simulink model "MEEN_432_Proj4Part2_version2025A"  (R2025a)
settings: Solver=VariableStepAuto  StartTime=0.0  StopTime=3600  FixedStep=0.01  RelTol=1e-3
undefined symbols (not defined in the file): carData, datBat, datCar, datMotor
libraries: slpidlib x1
settings Model: Creator=dxego  LastModifiedBy=jthin
settings OptimizationCC: ReuseModelBlockBuffer=off
settings RTWCC: GPUComputeCapability=3.5

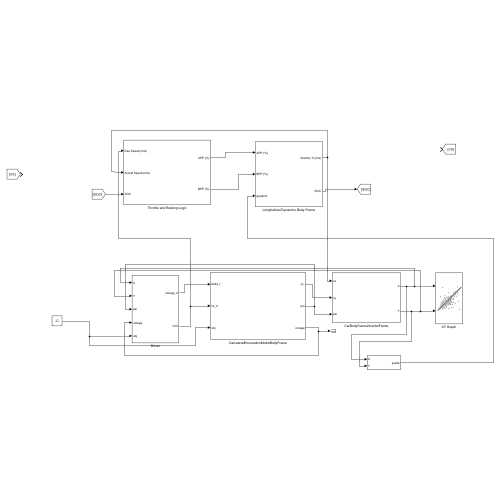
[thumbnail: Simulink's stored preview of the top-level diagram]
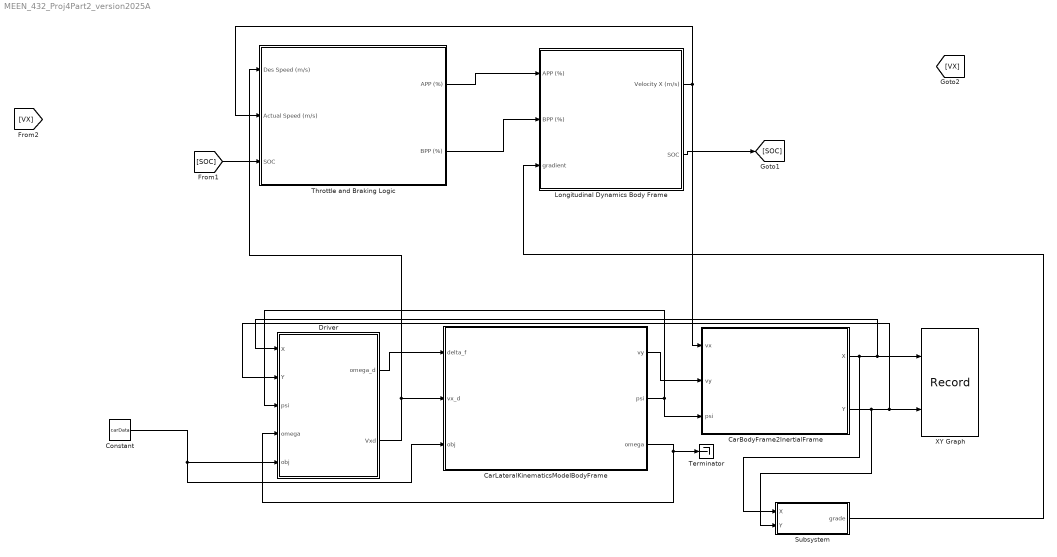
== system MEEN_432_Proj4Part2_version2025A ==
  CarBodyFrame2InertialFrame : Subsystem
  CarLateralKinematicsModelBodyFrame : Subsystem
  Constant : Constant  Value=carData  OutDataTypeStr=Bus: slBus1
  Driver : Subsystem
  Longitudinal Dynamics Body Frame : Subsystem
  Subsystem : Subsystem
  Terminator : Terminator
  "Throttle and Braking Logic " : Subsystem
  XY Graph : Record  NumPorts=2.0  FileSettingsInternal="{\"entries\":[{\"content\":{\"excelSettings\":{\"content\":{},\"type\":\"Streamout.ExcelSettings\"},\"parquetSettings\":{\"content\":{},\"type\":\"Streamout.ParquetSettings\"}},\"type\":\"Streamout.FileSettingStorage\",\"uuid\":\"\"}],\"packageUris\":[\"http:\\/\\/schema.mathworks.com\\/mf0\\/streamout_blocks\\/R2020a\"],\"version\":\"1.0\"}"  FrameSettings=[0, 0]  Layout=[1 1]  SignalsInternal="{\"entries\":[{\"content\":{\"signals\":[{\"content\":{\"blockPath\":[],\"dimensions\":[1],\"domain\":\"\",\"lineColor\":\"#a2142f\",\"plots\":[ 1 ],\"port\":1,\"signalID\":1,\"signalName\":\"CarBodyFrame2InertialFrame:1\"},\"type\":\"RecordBlkView.Signal\",\"uuid\":\"\"},{\"content\":{\"blockPath\":[],\"dimensions\":[1],\"domain\":\"\",\"lineColor\":\"#139fff\",\"plots\":[ 1 ],\"port\":2,\"signalID\":2,\"signalName\":\"CarBodyFrame2InertialFrame:2\"},\"type\":\"RecordBlkView.Signal\",\"uuid\":\"\"}]},\"type\":\"RecordBlkView.InputSignals\",\"uuid\":\"\"}],\"packageUris\":[\"http:\\/\\/schema.mathworks.com\\/mf0\\/streamout_blocks\\/R2020a\"],\"version\":\"1.0\"}"  VisualizationBindings="{\"xyplotplugin\":{\"info\":[{\"series\":[{\"bindingParametersList\":[{\"parameter\":\"X-Axis\",\"signalID\":1,\"signalName\":\"CarBodyFrame2InertialFrame:1\"},{\"parameter\":\"Y-Axis\",\"signalID\":2,\"signalName\":\"CarBodyFrame2InertialFrame:2\"}],\"seriesID\":0}],\"subplotID\":1}]}}"  CompatibilityTag=XY  st=-1
  wires:
  "Throttle and Braking Logic "/1(APP (%)) -> Longitudinal Dynamics Body Frame/1(APP (%))
  "Throttle and Braking Logic "/2(BPP (%)) -> Longitudinal Dynamics Body Frame/2("BPP (%) ")
  Longitudinal Dynamics Body Frame/2(SOC) -> [SOC]
  [SOC] -> "Throttle and Braking Logic "/3(SOC)
  CarLateralKinematicsModelBodyFrame/1("vy ") -> CarBodyFrame2InertialFrame/2(vy)
  Driver/1(omega_d) -> CarLateralKinematicsModelBodyFrame/1(delta_f)
  Constant/1 -> CarLateralKinematicsModelBodyFrame/3(obj), Driver/5(obj)
  CarBodyFrame2InertialFrame/2(Y) -> Subsystem/2(Y), Driver/2(Y), XY Graph/2
  CarLateralKinematicsModelBodyFrame/2(psi) -> CarBodyFrame2InertialFrame/3(psi), Driver/3(psi)
  CarBodyFrame2InertialFrame/1(X) -> Subsystem/1(X), Driver/1(X), XY Graph/1
  CarLateralKinematicsModelBodyFrame/3(omega) -> Driver/4(omega), Terminator/1
  Driver/2(Vxd) -> "Throttle and Braking Logic "/1("Des Speed (m/s) "), CarLateralKinematicsModelBodyFrame/2("vx_d ")
  Longitudinal Dynamics Body Frame/1(Velocity X (m/s)) -> "Throttle and Braking Logic "/2(Actual Speed (m/s)), CarBodyFrame2InertialFrame/1(vx)
  Subsystem/1(grade) -> Longitudinal Dynamics Body Frame/3(gradient)

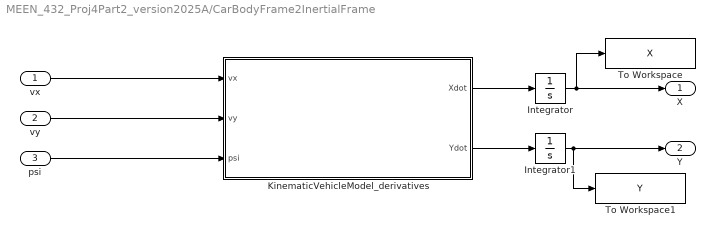
== system MEEN_432_Proj4Part2_version2025A/CarBodyFrame2InertialFrame ==
  vx : Inport
  vy : Inport  Port=2
  psi : Inport  Port=3
  Integrator : Integrator  InitialCondition=carData.init.X0
  Integrator1 : Integrator  InitialCondition=carData.init.Y0
  KinematicVehicleModel_derivatives : MATLAB Function  TreatAsAtomicUnit=on
  To Workspace : ToWorkspace  VariableName=X  SaveFormat=Timeseries  SampleTime=-1
  To Workspace1 : ToWorkspace  VariableName=Y  SaveFormat=Timeseries  SampleTime=-1
  X : Outport
  Y : Outport  Port=2
  wires:
  KinematicVehicleModel_derivatives/1(Xdot) -> Integrator/1
  KinematicVehicleModel_derivatives/2(Ydot) -> Integrator1/1
  Integrator/1 -> To Workspace/1, X/1
  Integrator1/1 -> To Workspace1/1, Y/1
  vx/1 -> KinematicVehicleModel_derivatives/1(vx)
  vy/1 -> KinematicVehicleModel_derivatives/2(vy)
  psi/1 -> KinematicVehicleModel_derivatives/3(psi)

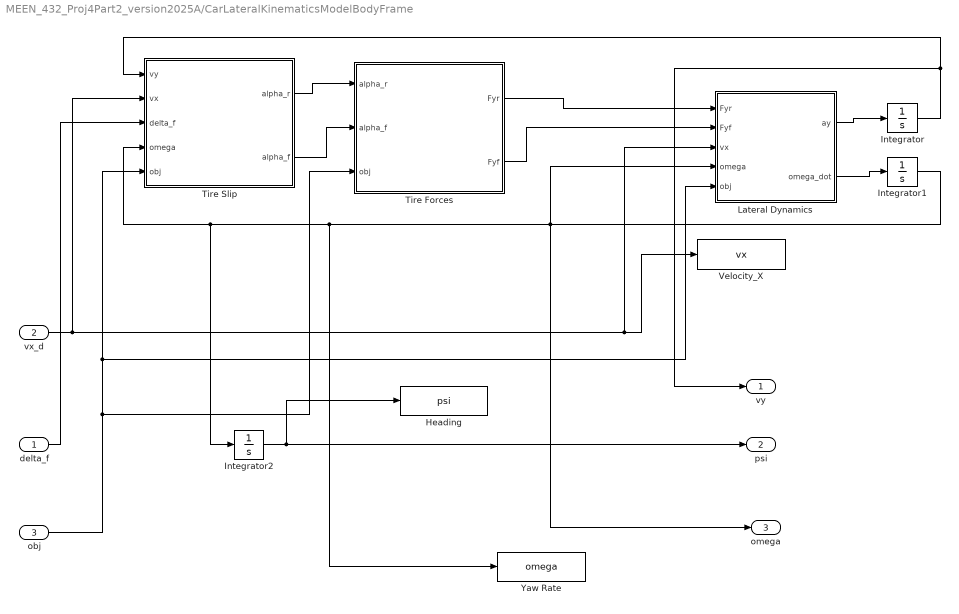
== system MEEN_432_Proj4Part2_version2025A/CarLateralKinematicsModelBodyFrame ==
  delta_f : Inport
  "vx_d " : Inport  Port=2
  obj : Inport  Port=3
  Heading : ToWorkspace  VariableName=psi  SaveFormat=Timeseries  SampleTime=-1
  Integrator : Integrator
  Integrator1 : Integrator
  Integrator2 : Integrator
  Lateral Dynamics : MATLAB Function  TreatAsAtomicUnit=on
  Tire Forces : MATLAB Function  TreatAsAtomicUnit=on
  Tire Slip : MATLAB Function  TreatAsAtomicUnit=on
  Velocity_X : ToWorkspace  VariableName=vx  SaveFormat=Timeseries  SampleTime=-1
  Yaw Rate : ToWorkspace  VariableName=omega  SaveFormat=Timeseries  SampleTime=-1
  "vy " : Outport
  psi : Outport  Port=2
  omega : Outport  Port=3
  wires:
  Integrator2/1 -> psi/1, Heading/1
  "vx_d "/1 -> Tire Slip/2(vx), Velocity_X/1, Lateral Dynamics/3(vx)
  delta_f/1 -> Tire Slip/3(delta_f)
  Integrator/1 -> "vy "/1, Tire Slip/1(vy)
  Tire Slip/1(alpha_r) -> Tire Forces/1(alpha_r)
  Tire Slip/2(alpha_f) -> Tire Forces/2(alpha_f)
  Lateral Dynamics/1(ay) -> Integrator/1
  Lateral Dynamics/2(omega_dot) -> Integrator1/1
  Integrator1/1 -> omega/1, Lateral Dynamics/4(omega), Yaw Rate/1, Integrator2/1, Tire Slip/4(omega)
  Tire Forces/1(Fyr) -> Lateral Dynamics/1(Fyr)
  Tire Forces/2(Fyf) -> Lateral Dynamics/2(Fyf)
  obj/1 -> Tire Forces/3(obj), Lateral Dynamics/5(obj), Tire Slip/5(obj)

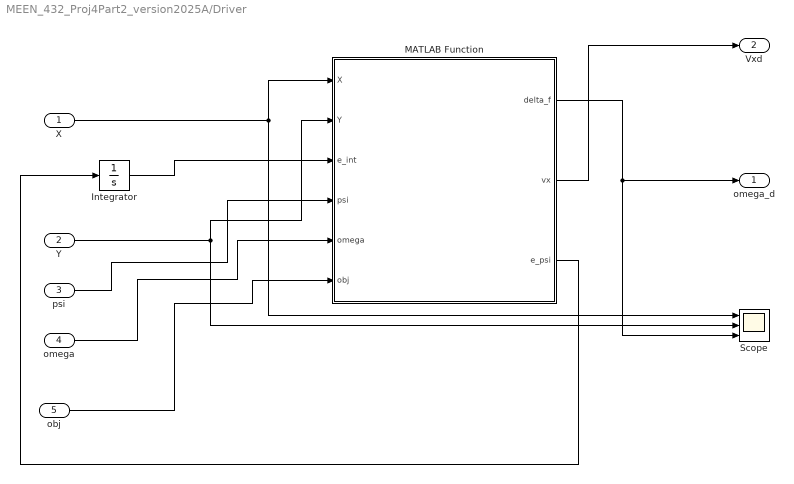
== system MEEN_432_Proj4Part2_version2025A/Driver ==
  X : Inport
  Y : Inport  Port=2
  psi : Inport  Port=3
  omega : Inport  Port=4
  obj : Inport  Port=5
  Integrator : Integrator
  MATLAB Function : MATLAB Function  TreatAsAtomicUnit=on
  Scope : Scope  NumInputPorts=3
      settings: ActiveDisplayYMinimum=-351.50186  ActiveDisplayYMaximum=1255.09761
  omega_d : Outport
  Vxd : Outport  Port=2
  wires:
  MATLAB Function/1(delta_f) -> omega_d/1, Scope/3
  MATLAB Function/2(vx) -> Vxd/1
  X/1 -> Scope/1, MATLAB Function/1(X)
  Y/1 -> Scope/2, MATLAB Function/2(Y)
  omega/1 -> MATLAB Function/5(omega)
  obj/1 -> MATLAB Function/6(obj)
  psi/1 -> MATLAB Function/4(psi)
  Integrator/1 -> MATLAB Function/3(e_int)
  MATLAB Function/3(e_psi) -> Integrator/1

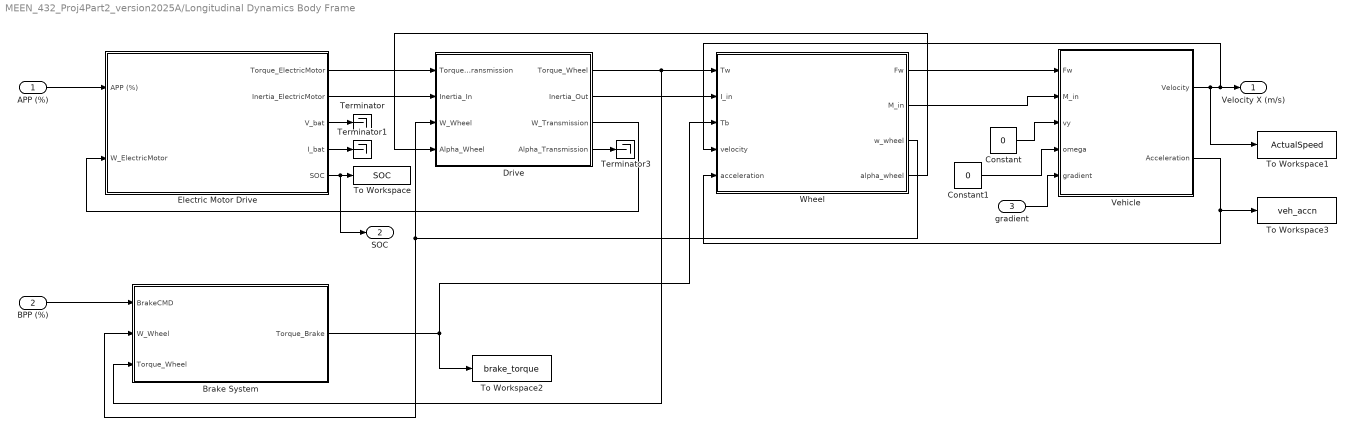
== system MEEN_432_Proj4Part2_version2025A/Longitudinal Dynamics Body Frame ==
  APP (%) : Inport
  "BPP (%) " : Inport  Port=2
  gradient : Inport  Port=3
  Brake System : Subsystem
  Constant : Constant  Value=0
  Constant1 : Constant  Value=0
  Drive : Subsystem
  Electric Motor Drive : Subsystem
  Terminator : Terminator
  Terminator1 : Terminator
  Terminator3 : Terminator
  To Workspace : ToWorkspace  VariableName=SOC  SaveFormat=Timeseries  SampleTime=-1
  To Workspace1 : ToWorkspace  VariableName=ActualSpeed  SaveFormat=Timeseries  SampleTime=-1
  To Workspace2 : ToWorkspace  VariableName=brake_torque  SaveFormat=Timeseries  SampleTime=-1
  To Workspace3 : ToWorkspace  VariableName=veh_accn  SaveFormat=Timeseries  SampleTime=-1
  Vehicle : Subsystem
  "Wheel " : Subsystem
  Velocity X (m/s) : Outport
  SOC : Outport  Port=2
  wires:
  Drive/3(W_Transmission) -> Electric Motor Drive/2(W_ElectricMotor)
  Electric Motor Drive/2(Inertia_ElectricMotor) -> Drive/2(Inertia_In)
  Electric Motor Drive/3(V_bat) -> Terminator/1
  Vehicle/2(Acceleration) -> "Wheel "/5(acceleration), To Workspace3/1
  Drive/1(Torque_Wheel) -> "Wheel "/1(Tw), Brake System/3(Torque_Wheel)
  Electric Motor Drive/1(Torque_ElectricMotor) -> Drive/1(Torque_Transmission)
  Drive/2(Inertia_Out) -> "Wheel "/2(I_in)
  "Wheel "/2(M_in) -> Vehicle/2("M_in ")
  "BPP (%) "/1 -> Brake System/1("BrakeCMD ")
  "Wheel "/3(w_wheel) -> Brake System/2(W_Wheel), Drive/3(W_Wheel)
  "Wheel "/1(Fw) -> Vehicle/1("Fw ")
  Brake System/1(Torque_Brake) -> To Workspace2/1, "Wheel "/3(Tb)
  Drive/4(Alpha_Transmission) -> Terminator3/1
  "Wheel "/4(alpha_wheel) -> Drive/4(Alpha_Wheel)
  Electric Motor Drive/4(I_bat) -> Terminator1/1
  APP (%)/1 -> Electric Motor Drive/1(APP (%))
  Constant/1 -> Vehicle/3(vy)
  Constant1/1 -> Vehicle/4(omega)
  Vehicle/1("Velocity ") -> To Workspace1/1, "Wheel "/4(velocity), Velocity X (m/s)/1
  Electric Motor Drive/5(SOC) -> SOC/1, To Workspace/1
  gradient/1 -> Vehicle/5(gradient)

== system MEEN_432_Proj4Part2_version2025A/Subsystem ==
  X : Inport
  Y : Inport  Port=2
  MATLAB Function : MATLAB Function  TreatAsAtomicUnit=on
  grade : Outport
  wires:
  X/1 -> MATLAB Function/1(X)
  Y/1 -> MATLAB Function/2(Y)
  MATLAB Function/1(calculate_gradient) -> grade/1

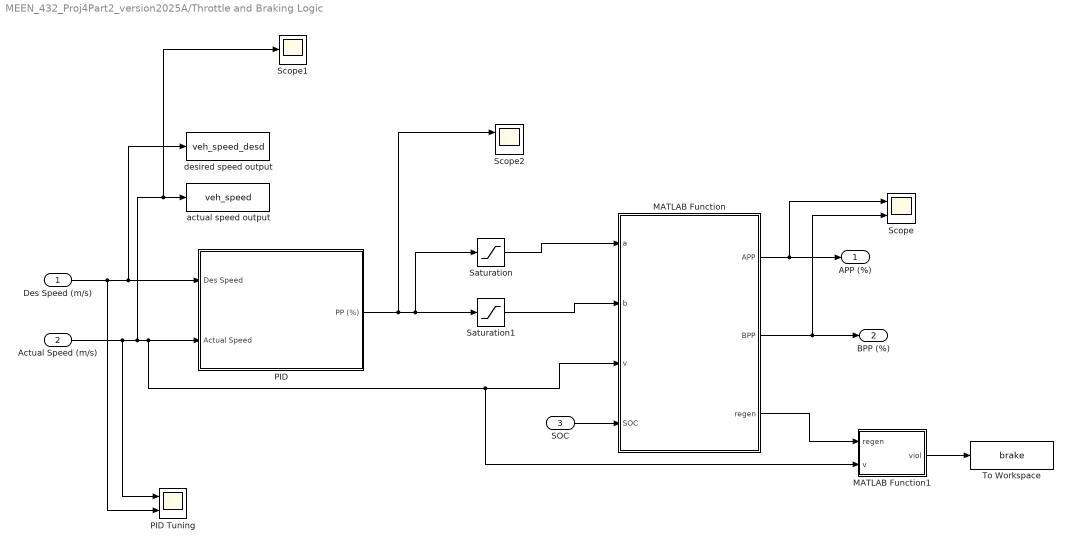
== system MEEN_432_Proj4Part2_version2025A/Throttle and Braking Logic  ==
  "Des Speed (m/s) " : Inport
  Actual Speed (m/s) : Inport  Port=2
  SOC : Inport  Port=3
  MATLAB Function : MATLAB Function  TreatAsAtomicUnit=on
  MATLAB Function1 : MATLAB Function  TreatAsAtomicUnit=on
  PID : Subsystem
  PID Tuning : Scope  NumInputPorts=2
      settings: ActiveDisplayYMinimum=-4.40832  ActiveDisplayYMaximum=37.63006
  Saturation : Saturate  UpperLimit=1  LowerLimit=0
  Saturation1 : Saturate  UpperLimit=0  LowerLimit=-1
  Scope : Scope  NumInputPorts=2
      settings: ActiveDisplayYMinimum=-1.0607  ActiveDisplayYMaximum=1.06103
  Scope1 : Scope
      settings: ActiveDisplayYMinimum=-3.08288  ActiveDisplayYMaximum=27.75461
  Scope2 : Scope  NumInputPorts=2
      settings: ActiveDisplayYMinimum=-1.0607  ActiveDisplayYMaximum=1.06103  DataLoggingVariableName=ScopeData5
  To Workspace : ToWorkspace  VariableName=brake  SaveFormat=Timeseries  SampleTime=-1
  actual speed output : ToWorkspace  VariableName=veh_speed  SaveFormat=Timeseries  SampleTime=-1
  desired speed output : ToWorkspace  VariableName=veh_speed_desd  SaveFormat=Timeseries  SampleTime=-1
  APP (%) : Outport
  BPP (%) : Outport  Port=2
  wires:
  PID/1(PP (%)) -> Scope2/1, Saturation1/1, Saturation/1
  Saturation1/1 -> MATLAB Function/2(b)
  Actual Speed (m/s)/1 -> PID Tuning/1, Scope1/1, actual speed output/1, MATLAB Function1/2(v), MATLAB Function/3(v), PID/2(Actual Speed)
  "Des Speed (m/s) "/1 -> PID Tuning/2, desired speed output/1, PID/1("Des Speed ")
  Saturation/1 -> MATLAB Function/1(a)
  MATLAB Function/1(APP) -> Scope/1, APP (%)/1
  MATLAB Function/2(BPP) -> Scope/2, BPP (%)/1
  MATLAB Function1/1(viol) -> To Workspace/1
  SOC/1 -> MATLAB Function/4(SOC)
  MATLAB Function/3(regen) -> MATLAB Function1/1(regen)

== system MEEN_432_Proj4Part2_version2025A/Longitudinal Dynamics Body Frame/Brake System ==
  "BrakeCMD " : Inport
  W_Wheel : Inport  Port=2
  Torque_Wheel : Inport  Port=3
  Brake Torque : MATLAB Function  TreatAsAtomicUnit=on
  Constant : Constant  Value=datCar.maxBrakeTorque
  Scope : Scope
      settings: ActiveDisplayYMinimum=-3252.17168  ActiveDisplayYMaximum=56.62718  DataLoggingVariableName=ScopeData4
  Torque_Brake : Outport  VectorParamsAs1DForOutWhenUnconnected=off
  wires:
  "BrakeCMD "/1 -> Brake Torque/1(BBcmd)
  Brake Torque/1(Tb) -> Scope/1, Torque_Brake/1
  W_Wheel/1 -> Brake Torque/3(w_wheel)
  Constant/1 -> Brake Torque/2(Tbcap)

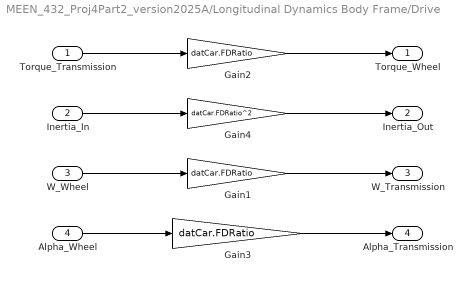
== system MEEN_432_Proj4Part2_version2025A/Longitudinal Dynamics Body Frame/Drive ==
  Torque_Transmission : Inport
  Inertia_In : Inport  Port=2
  W_Wheel : Inport  Port=3
  Alpha_Wheel : Inport  Port=4
  Gain1 : Gain  Gain=datCar.FDRatio
  Gain2 : Gain  Gain=datCar.FDRatio
  Gain3 : Gain  Gain=datCar.FDRatio
  Gain4 : Gain  Gain=datCar.FDRatio^2
  Torque_Wheel : Outport
  Inertia_Out : Outport  Port=2
  W_Transmission : Outport  Port=3
  Alpha_Transmission : Outport  Port=4
  wires:
  Torque_Transmission/1 -> Gain2/1
  Gain2/1 -> Torque_Wheel/1
  Inertia_In/1 -> Gain4/1
  Gain4/1 -> Inertia_Out/1
  W_Wheel/1 -> Gain1/1
  Gain1/1 -> W_Transmission/1
  Alpha_Wheel/1 -> Gain3/1
  Gain3/1 -> Alpha_Transmission/1

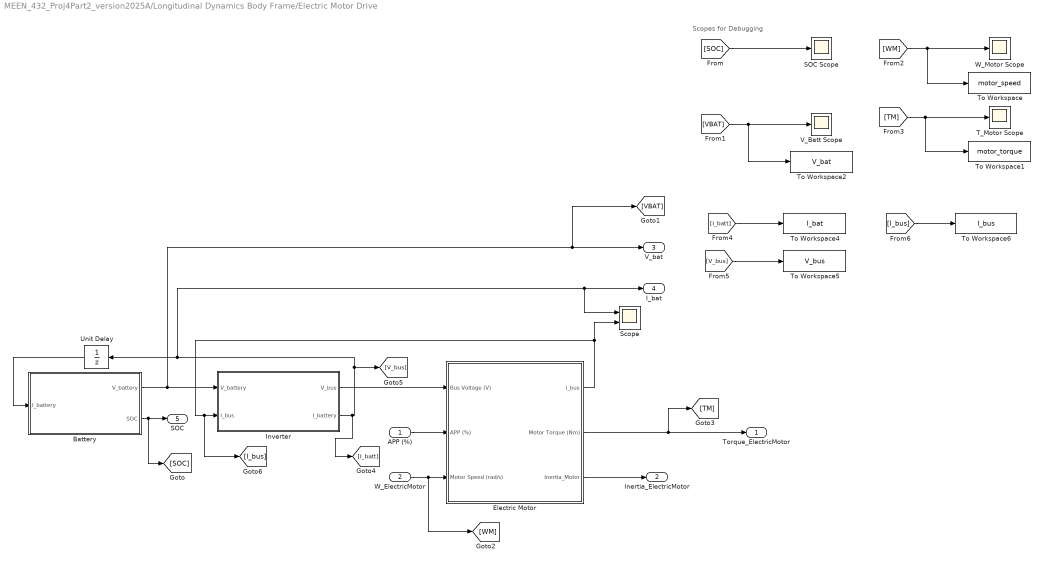
== system MEEN_432_Proj4Part2_version2025A/Longitudinal Dynamics Body Frame/Electric Motor Drive ==
  note: Scopes for Debugging
  APP (%) : Inport
  W_ElectricMotor : Inport  Port=2
  Battery : Subsystem
  Electric Motor : Subsystem
  Inverter : Subsystem
  SOC Scope : Scope
      settings: ActiveDisplayYMinimum=0.79068  ActiveDisplayYMaximum=0.80103  DataLoggingVariableName=ScopeData7
  Scope : Scope  NumInputPorts=2
      settings: ActiveDisplayYMinimum=-92.41521  ActiveDisplayYMaximum=118.26537  DataLoggingVariableName=ScopeData2
  T_Motor Scope : Scope
      settings: ActiveDisplayYMinimum=-92.74121  ActiveDisplayYMaximum=115.47111  DataLoggingVariableName=ScopeData10
  To Workspace : ToWorkspace  VariableName=motor_speed  SaveFormat=Timeseries  SampleTime=-1
  To Workspace1 : ToWorkspace  VariableName=motor_torque  SaveFormat=Timeseries  SampleTime=-1
  To Workspace2 : ToWorkspace  VariableName=V_bat  SaveFormat=Timeseries  SampleTime=-1
  To Workspace4 : ToWorkspace  VariableName=I_bat  SaveFormat=Timeseries  SampleTime=-1
  To Workspace5 : ToWorkspace  VariableName=V_bus  SaveFormat=Timeseries  SampleTime=-1
  To Workspace6 : ToWorkspace  VariableName=I_bus  SaveFormat=Timeseries  SampleTime=-1
  Unit Delay : UnitDelay  SampleTime=-1  HasFrameUpgradeWarning=on
  V_Batt Scope : Scope
      settings: ActiveDisplayYMinimum=354.15627  ActiveDisplayYMaximum=391.49042  DataLoggingVariableName=ScopeData8
  W_Motor Scope : Scope
      settings: ActiveDisplayYMinimum=-83.74997  ActiveDisplayYMaximum=695.87961  DataLoggingVariableName=ScopeData9
  Torque_ElectricMotor : Outport
  Inertia_ElectricMotor : Outport  Port=2
  V_bat : Outport  Port=3
  I_bat : Outport  Port=4
  SOC : Outport  Port=5
  wires:
  APP (%)/1 -> Electric Motor/2(APP (%))
  W_ElectricMotor/1 -> [WM], Electric Motor/3(Motor Speed (rad/s))
  Electric Motor/3(Inertia_Motor) -> Inertia_ElectricMotor/1
  Inverter/1(V_bus) -> Electric Motor/1(Bus Voltage (V))
  Inverter/2(I_battery) -> [I_batt], Scope/1, I_bat/1, Unit Delay/1, [V_bus]
  Electric Motor/1(I_bus) -> Scope/2, [I_bus], Inverter/2(I_bus)
  [SOC] -> SOC Scope/1
  [VBAT] -> To Workspace2/1, V_Batt Scope/1
  [WM] -> To Workspace/1, W_Motor Scope/1
  [TM] -> To Workspace1/1, T_Motor Scope/1
  Battery/1(V_battery) -> [VBAT], V_bat/1, Inverter/1(V_battery)
  Electric Motor/2(Motor Torque (Nm)) -> [TM], Torque_ElectricMotor/1
  Battery/2(SOC) -> [SOC], SOC/1
  [I_batt] -> To Workspace4/1
  [V_bus] -> To Workspace5/1
  [I_bus] -> To Workspace6/1
  Unit Delay/1 -> Battery/1(I_battery)

== system MEEN_432_Proj4Part2_version2025A/Longitudinal Dynamics Body Frame/Vehicle ==
  "Fw " : Inport
  "M_in " : Inport  Port=2
  vy : Inport  Port=3
  omega : Inport  Port=4
  gradient : Inport  Port=5
  vehicleDragForce : Subsystem
  vehicleDynamics : Subsystem
  "Velocity " : Outport  VectorParamsAs1DForOutWhenUnconnected=off
  Acceleration : Outport  Port=2
  wires:
  vehicleDynamics/2(Out2) -> vehicleDragForce/1(vel), "Velocity "/1
  "Fw "/1 -> vehicleDynamics/1("Fw ")
  vehicleDragForce/1(Fdrag) -> vehicleDynamics/2(Fd)
  "M_in "/1 -> vehicleDynamics/3("M_in ")
  vy/1 -> vehicleDynamics/4(vy)
  omega/1 -> vehicleDynamics/5(omega)
  vehicleDynamics/1(acceleration) -> Acceleration/1
  gradient/1 -> vehicleDynamics/6(gradient)

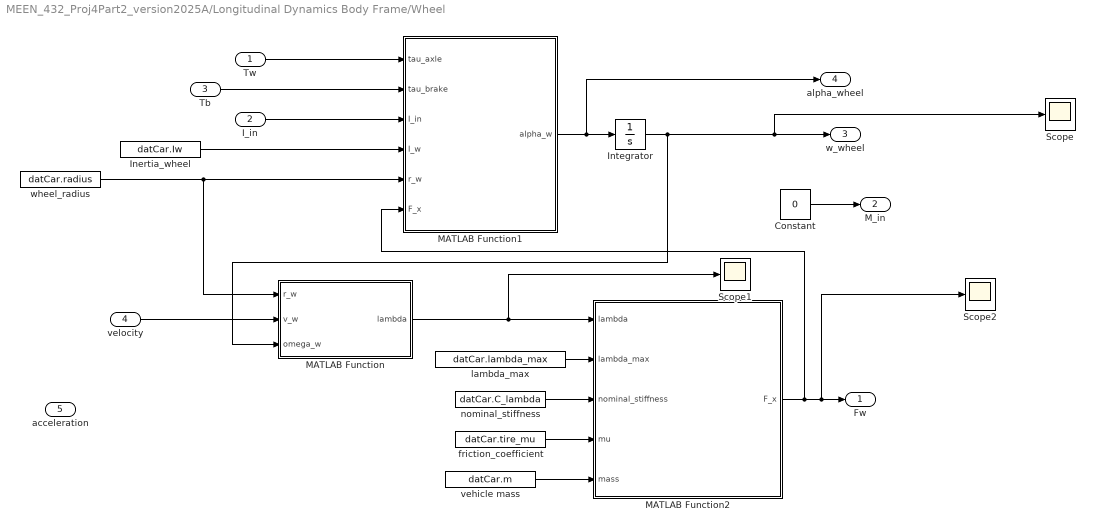
== system MEEN_432_Proj4Part2_version2025A/Longitudinal Dynamics Body Frame/Wheel  ==
  Tw : Inport
  I_in : Inport  Port=2
  Tb : Inport  Port=3
  velocity : Inport  Port=4
  acceleration : Inport  Port=5
  Constant : Constant  Value=0
  Inertia_wheel : Constant  Value=datCar.Iw
  Integrator : Integrator  InitialCondition=datCar.init.omega0
  MATLAB Function : MATLAB Function  TreatAsAtomicUnit=on
  MATLAB Function1 : MATLAB Function  TreatAsAtomicUnit=on
  MATLAB Function2 : MATLAB Function  TreatAsAtomicUnit=on
  Scope : Scope
      settings: ActiveDisplayYMinimum=-11.16666  ActiveDisplayYMaximum=92.78395
  Scope1 : Scope
      settings: ActiveDisplayYMinimum=-33.74112  ActiveDisplayYMaximum=2.76989  DataLoggingVariableName=ScopeData2
  Scope2 : Scope
      settings: ActiveDisplayYMinimum=-88.22724  ActiveDisplayYMaximum=2.56826  DataLoggingVariableName=ScopeData3
  friction_coefficient : Constant  Value=datCar.tire_mu
  lambda_max : Constant  Value=datCar.lambda_max
  nominal_stiffness : Constant  Value=datCar.C_lambda
  vehicle mass : Constant  Value=datCar.m
  wheel_radius : Constant  Value=datCar.radius
  Fw : Outport
  M_in : Outport  Port=2
  w_wheel : Outport  Port=3
  alpha_wheel : Outport  Port=4
  wires:
  velocity/1 -> MATLAB Function/2(v_w)
  Tw/1 -> MATLAB Function1/1(tau_axle)
  Tb/1 -> MATLAB Function1/2(tau_brake)
  I_in/1 -> MATLAB Function1/3(I_in)
  Inertia_wheel/1 -> MATLAB Function1/4(I_w)
  wheel_radius/1 -> MATLAB Function/1(r_w), MATLAB Function1/5(r_w)
  MATLAB Function1/1(alpha_w) -> Integrator/1, alpha_wheel/1
  Integrator/1 -> MATLAB Function/3(omega_w), Scope/1, w_wheel/1
  MATLAB Function/1(lambda) -> Scope1/1, MATLAB Function2/1(lambda)
  nominal_stiffness/1 -> MATLAB Function2/3(nominal_stiffness)
  lambda_max/1 -> MATLAB Function2/2(lambda_max)
  friction_coefficient/1 -> MATLAB Function2/4(mu)
  vehicle mass/1 -> MATLAB Function2/5(mass)
  MATLAB Function2/1(F_x) -> Scope2/1, Fw/1, MATLAB Function1/6(F_x)
  Constant/1 -> M_in/1

== system MEEN_432_Proj4Part2_version2025A/Throttle and Braking Logic /PID ==
  "Des Speed " : Inport
  Actual Speed : Inport  Port=2
  PID Controller : slpidlib/PID Controller  Controller=PID  Form=Parallel  TimeDomain=Continuous-time  UseExternalTs=off  SampleTime=-1  IntegratorMethod=Forward Euler  FilterMethod=Forward Euler  ControllerParametersSource=internal  P=0.3  I=0  UseKiTs=off  D=0  UseExternalDerivativeSource=off  N=100  UseFilter=on  TunerSelectOption=Transfer Function Based (PID Tuner App)  InitialConditionSource=internal  InitialConditionForIntegrator=0  InitialConditionForFilter=0  DifferentiatorICPrevScaledInput=0  ExternalReset=none  TrackingMode=off  Kt=1  LimitOutput=off  SatLimitsSource=internal  UpperSaturationLimit=inf  LowerSaturationLimit=-inf  LinearizeAsGain=on  AntiWindupMode=none  Kb=1  LimitIntegrator=off  UpperIntegratorSaturationLimit=inf  LowerIntegratorSaturationLimit=-inf  POutMin=[]  POutMax=[]  IOutMin=[]  IOutMax=[]  DOutMin=[]  DOutMax=[]  NOutMin=[]  NOutMax=[]  SumOutMin=[]  SumOutMax=[]  SaturationOutMin=[]  SaturationOutMax=[]  PParamMin=[]  PParamMax=[]  IParamMin=[]  IParamMax=[]  DParamMin=[]  DParamMax=[]  NParamMin=[]  NParamMax=[]  KbParamMin=[]  KbParamMax=[]  KtParamMin=[]  KtParamMax=[]  KbOutMin=[]  KbOutMax=[]  KtOutMin=[]  KtOutMax=[]  IntegratorOutMin=[]  IntegratorOutMax=[]  FilterOutMin=[]  FilterOutMax=[]  SumI1OutMin=[]  SumI1OutMax=[]  SumI2OutMin=[]  SumI2OutMax=[]  SumI3OutMin=[]  SumI3OutMax=[]  SumI4OutMin=[]  SumI4OutMax=[]  SumDOutMin=[]  SumDOutMax=[]  DifferentiatorOutMin=[]  DifferentiatorOutMax=[]  FilterDiffOutCoefMin=[]  FilterDiffOutCoefMax=[]  ReciprocalOutMin=[]  ReciprocalOutMax=[]  SumDenOutMin=[]  SumDenOutMax=[]  SumNumOutMin=[]  SumNumOutMax=[]  DivideOutMin=[]  DivideOutMax=[]  UdiffTsProdOutMin=[]  UdiffTsProdOutMax=[]  NTsProdOutMin=[]  NTsProdOutMax=[]  UintegralTsProdOutMin=[]  UintegralTsProdOutMax=[]  UngainTsProdOutMin=[]  UngainTsProdOutMax=[]  ClampingZeroOutDataTypeStr=Inherit: Inherit via back propagation  ClampingZeroOutMin=[]  ClampingZeroOutMax=[]  FilterDenConstantOutDataTypeStr=Inherit: Inherit via back propagation  FilterDenConstantOutMin=[]  FilterDenConstantOutMax=[]  PCopyOutDataTypeStr=Inherit: Inherit via back propagation  PCopyOutMin=[]  PCopyOutMax=[]  NCopyOutDataTypeStr=Inherit: Inherit via back propagation  NCopyOutMin=[]  NCopyOutMax=[]  IntegratorContinuousStateAttributes=''  IntegratorStateMustResolveToSignalObject=off  IntegratorRTWStateStorageClass=Auto  FilterContinuousStateAttributes=''  FilterStateMustResolveToSignalObject=off  FilterRTWStateStorageClass=Auto  ParallelPVariant=InternalParameters  IdealPVariant=Disabled  IVariant=InternalParameters  DVariant=InternalParameters  IntegratorVariant=Continuous  SatVariant=Disabled  AWVariant=Passthrough  PCopyVariant=Disabled  TRVariant=Disabled  FdbkBlocksVariant=Forward  IdealPFdbkVariant=Disabled  SatFdbkVariant=Disabled  DerivativeFilterVariant=ContFilter  NVariant=InternalParameters  NCopyVariant=Disabled  FilterICVariant=InternalICsFilter  IntegratorICVariant=InternalICs  ExternalResetVariant=Disabled  TRSumVariant=Passthrough  SumFdbkVariant=Disabled  SumVariant=Sum_PID  TsampFilterVariant=InternalTs  TsampNgainVariant=Passthrough  TsampIntegralVariant=Disabled_SignalSpec  ExternalSaturationOutDataTypeStr=Inherit: Same as second input  DerivativeSourceVariant=ErrorSignal  PreIntVariant=InternalPreInt
  Sum : Sum  Inputs=|+-
  To Workspace : ToWorkspace  VariableName=v_error  SaveFormat=Timeseries  SampleTime=-1
  PP (%) : Outport
  wires:
  Sum/1 -> PID Controller/1, To Workspace/1
  "Des Speed "/1 -> Sum/1
  Actual Speed/1 -> Sum/2
  PID Controller/1 -> PP (%)/1

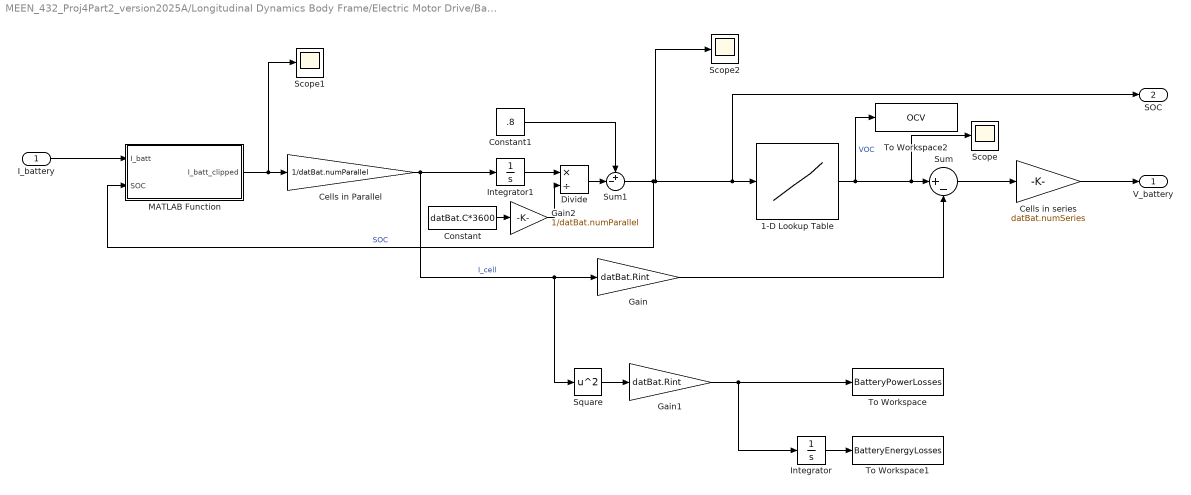
== system MEEN_432_Proj4Part2_version2025A/Longitudinal Dynamics Body Frame/Electric Motor Drive/Battery ==
  I_battery : Inport
  1-D Lookup Table : Lookup_n-D  NumberOfTableDimensions=1  BreakpointsForDimension1=datBat.SOC  Table=datBat.OCV  ExtrapMethod=Clip  UseLastTableValue=on  InternalRulePriority=Speed  RndMeth=Simplest
  Cells in Parallel : Gain  Gain=1/datBat.numParallel
  Cells in series : Gain  Gain=datBat.numSeries
  Constant : Constant  Value=datBat.C*3600
  Constant1 : Constant  Value=.8
  Divide : Product  Inputs=*/
  Gain : Gain  Gain=datBat.Rint
  Gain1 : Gain  Gain=datBat.Rint
  Gain2 : Gain  Gain=1/datBat.numParallel
  Integrator : Integrator
  Integrator1 : Integrator  InitialCondition=1459.5
  MATLAB Function : MATLAB Function  TreatAsAtomicUnit=on
  Scope : Scope
      settings: ActiveDisplayYMinimum=3.9447746248567759  ActiveDisplayYMaximum=3.9505775108183836  DataLoggingVariableName=ScopeData5
  Scope1 : Scope
      settings: ActiveDisplayYMinimum=-38.071970075878966  ActiveDisplayYMaximum=120.71055450400272  DataLoggingVariableName=ScopeData6
  Scope2 : Scope
      settings: ActiveDisplayYMinimum=0.78954924829198925  ActiveDisplayYMaximum=0.80115502179471731
  Square : Math  Operator=square
  Sum : Sum  Inputs=|+-
  Sum1 : Sum  Inputs=+-|
  To Workspace : ToWorkspace  VariableName=BatteryPowerLosses  SaveFormat=Timeseries  SampleTime=-1
  To Workspace1 : ToWorkspace  VariableName=BatteryEnergyLosses  SaveFormat=Timeseries  SampleTime=-1
  To Workspace2 : ToWorkspace  VariableName=OCV  SaveFormat=Timeseries  SampleTime=-1
  V_battery : Outport
  SOC : Outport  Port=2
  wires:
  Cells in Parallel/1 -> Square/1, Gain/1, Integrator1/1  "I_cell"
  Sum1/1 -> MATLAB Function/2(SOC), SOC/1, 1-D Lookup Table/1, Scope2/1  "SOC"
  1-D Lookup Table/1 -> To Workspace2/1, Scope/1, Sum/1  "VOC"
  Gain/1 -> Sum/2
  Sum/1 -> Cells in series/1
  Cells in series/1 -> V_battery/1
  Integrator1/1 -> Divide/1
  Divide/1 -> Sum1/2
  Constant1/1 -> Sum1/1
  Square/1 -> Gain1/1
  Gain1/1 -> Integrator/1, To Workspace/1
  Integrator/1 -> To Workspace1/1
  Constant/1 -> Gain2/1
  Gain2/1 -> Divide/2
  I_battery/1 -> MATLAB Function/1(I_batt)
  MATLAB Function/1(I_batt_clipped) -> Scope1/1, Cells in Parallel/1

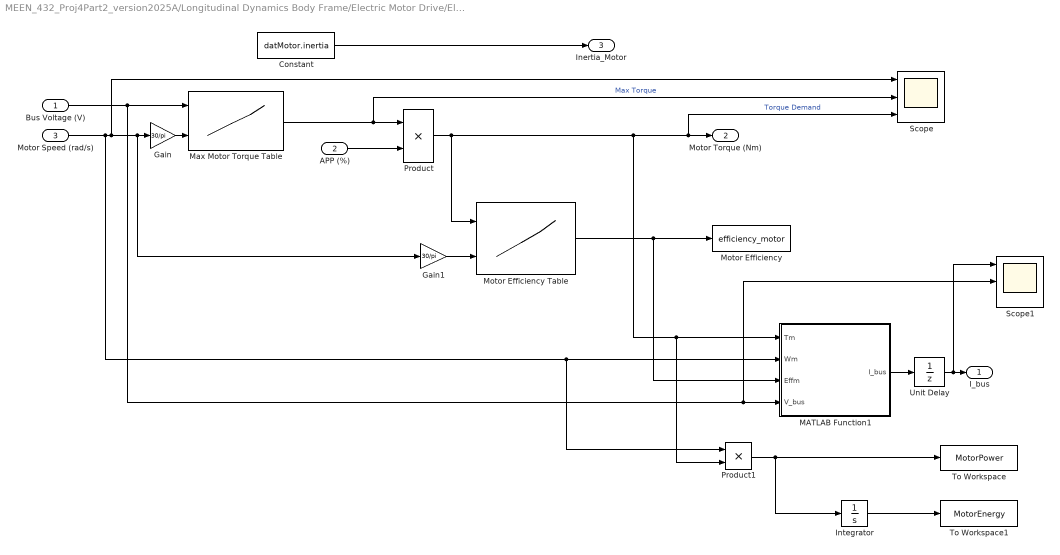
== system MEEN_432_Proj4Part2_version2025A/Longitudinal Dynamics Body Frame/Electric Motor Drive/Electric Motor ==
  Bus Voltage (V) : Inport
  APP (%) : Inport  Port=2
  Motor Speed (rad/s) : Inport  Port=3
  Constant : Constant  Value=datMotor.inertia
  Gain : Gain  Gain=30/pi
  Gain1 : Gain  Gain=30/pi
  Integrator : Integrator
  MATLAB Function1 : MATLAB Function  TreatAsAtomicUnit=on
  Max Motor Torque Table : Lookup_n-D  BreakpointsForDimension1=datMotor.vbus  BreakpointsForDimension2=datMotor.rpm  BreakpointsForDimension3=[5, 7]  Table=datMotor.maxtorque  ExtrapMethod=Clip  UseLastTableValue=on  InternalRulePriority=Speed  RndMeth=Simplest
      settings: InputPortMap=u0,u1
  Motor Efficiency : ToWorkspace  VariableName=efficiency_motor  SaveFormat=Timeseries  SampleTime=-1
  Motor Efficiency Table : Lookup_n-D  BreakpointsForDimension1=datMotor.eta_torque  BreakpointsForDimension2=datMotor.eta_speed  BreakpointsForDimension3=[5, 7]  Table=datMotor.eta_val  ExtrapMethod=Clip  UseLastTableValue=on  InternalRulePriority=Speed  RndMeth=Simplest
      settings: InputPortMap=u0,u1
  Product : Product
  Product1 : Product
  Scope : Scope  NumInputPorts=3
      settings: ActiveDisplayYMinimum=-117.53104  ActiveDisplayYMaximum=699.63306
  Scope1 : Scope  NumInputPorts=3
      settings: ActiveDisplayYMinimum=-70.21177  ActiveDisplayYMaximum=433.2973  DataLoggingVariableName=ScopeData2
  To Workspace : ToWorkspace  VariableName=MotorPower  SaveFormat=Timeseries  SampleTime=-1
  To Workspace1 : ToWorkspace  VariableName=MotorEnergy  SaveFormat=Timeseries  SampleTime=-1
  Unit Delay : UnitDelay  SampleTime=-1  HasFrameUpgradeWarning=on
  I_bus : Outport
  Motor Torque (Nm) : Outport  Port=2
  Inertia_Motor : Outport  Port=3
  wires:
  Max Motor Torque Table/1 -> Scope/2, Product/1  "Max Torque"
  Constant/1 -> Inertia_Motor/1
  APP (%)/1 -> Product/2
  Product/1 -> Product1/2, MATLAB Function1/1(Tm), Scope/3, Motor Torque (Nm)/1, Motor Efficiency Table/1  "Torque Demand"
  Motor Efficiency Table/1 -> Motor Efficiency/1, MATLAB Function1/3(Effm)
  MATLAB Function1/1(I_bus) -> Unit Delay/1
  Bus Voltage (V)/1 -> Scope1/2, MATLAB Function1/4(V_bus), Max Motor Torque Table/1
  Unit Delay/1 -> Scope1/1, I_bus/1
  Product1/1 -> Integrator/1, To Workspace/1
  Integrator/1 -> To Workspace1/1
  Gain/1 -> Max Motor Torque Table/2
  Gain1/1 -> Motor Efficiency Table/2
  Motor Speed (rad/s)/1 -> Product1/1, MATLAB Function1/2(Wm), Scope/1, Gain1/1, Gain/1

== system MEEN_432_Proj4Part2_version2025A/Longitudinal Dynamics Body Frame/Electric Motor Drive/Inverter ==
  V_battery : Inport
  I_bus : Inport  Port=2
  Efficiency Inverter : Constant  Value=0.95
  Inverter Calculations : MATLAB Function  TreatAsAtomicUnit=on
  V_bus : Outport
  I_battery : Outport  Port=2
  wires:
  V_battery/1 -> Inverter Calculations/1(V_bat)
  Inverter Calculations/1(V_bus) -> V_bus/1
  Efficiency Inverter/1 -> Inverter Calculations/2(Eff_I)
  I_bus/1 -> Inverter Calculations/3(I_bus)
  Inverter Calculations/2(I_bat) -> I_battery/1

== system MEEN_432_Proj4Part2_version2025A/Longitudinal Dynamics Body Frame/Vehicle/vehicleDragForce ==
  vel : Inport
  Drag Force : MATLAB Function  TreatAsAtomicUnit=on
  To Workspace : ToWorkspace  VariableName=Faero  SaveFormat=Timeseries  SampleTime=-1
  drag coeff : Constant  Value=datCar.C2
  rolling friction coeff : Constant  Value=datCar.C1
  static friction : Constant  Value=datCar.C0
  Fdrag : Outport
  wires:
  static friction/1 -> Drag Force/1(C0)
  Drag Force/1(Fdrag) -> Fdrag/1, To Workspace/1
  vel/1 -> Drag Force/4(vel)
  rolling friction coeff/1 -> Drag Force/2(C1)
  drag coeff/1 -> Drag Force/3(C2)

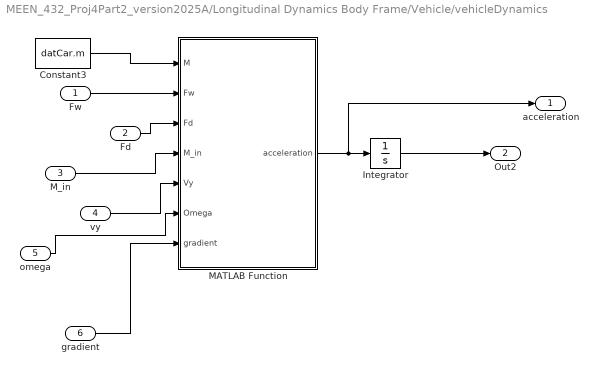
== system MEEN_432_Proj4Part2_version2025A/Longitudinal Dynamics Body Frame/Vehicle/vehicleDynamics ==
  "Fw " : Inport
  Fd : Inport  Port=2
  "M_in " : Inport  Port=3
  vy : Inport  Port=4
  omega : Inport  Port=5
  gradient : Inport  Port=6
  Constant3 : Constant  Value=datCar.m
  Integrator : Integrator  InitialCondition=datCar.init.vx0  LimitOutput=on  LowerSaturationLimit=0
  MATLAB Function : MATLAB Function  TreatAsAtomicUnit=on
  acceleration : Outport
  Out2 : Outport  Port=2
  wires:
  MATLAB Function/1(acceleration) -> acceleration/1, Integrator/1
  "Fw "/1 -> MATLAB Function/2(Fw)
  vy/1 -> MATLAB Function/5(Vy)
  "M_in "/1 -> MATLAB Function/4(M_in)
  Constant3/1 -> MATLAB Function/1(M)
  omega/1 -> MATLAB Function/6(Omega)
  Fd/1 -> MATLAB Function/3(Fd)
  Integrator/1 -> Out2/1
  gradient/1 -> MATLAB Function/7(gradient)

== matlab function MEEN_432_Proj4Part2_version2025A/Longitudinal Dynamics Body Frame/Vehicle/vehicleDragForce/Drag Force ==
  data: C0 input; Fdrag output; C1 input; C2 input; vel input
function Fdrag = drag(C0, C1, C2, vel)
    
Fdrag = C0 + C1*vel + C2*(vel)^2;

== matlab function MEEN_432_Proj4Part2_version2025A/Longitudinal Dynamics Body Frame/Vehicle/vehicleDynamics/MATLAB Function ==
  data: M input; Fw input; Fd input; acceleration output; M_in input; Vy input; Omega input; gradient input
function acceleration = vehicle(M, Fw, Fd, M_in, Vy, Omega, gradient)

g=9.8;
acceleration = ((Fw - Fd - M*g*sin(atan(gradient))) / (M + M_in)) + Vy*Omega;

== matlab function MEEN_432_Proj4Part2_version2025A/CarLateralKinematicsModelBodyFrame/Tire Forces ==
  data: Fyr output; Fyf output; alpha_r input; alpha_f input; obj input
function [Fyr, Fyf] = fcn(alpha_r, alpha_f, obj)


Fyr = obj.Calpha_r * alpha_r;
Fyf = obj.Calpha_f * alpha_f;

if abs(Fyr) > obj.Fyrmax
    Fyr = obj.Fyrmax*sign(Fyr);

end

if abs(Fyf) > obj.Fyfmax
    Fyf = obj.Fyfmax*sign(Fyf);

end

== matlab function MEEN_432_Proj4Part2_version2025A/Throttle and Braking Logic /MATLAB Function ==
  data: a input; APP output; b input; v input; BPP output; SOC input; regen output
function [APP, BPP, regen] = fcn(a, b, v, SOC)

    speed1 = 5*1600/3600;
    speed2 = 25*1600/3600;
    dspeed = speed2 - speed1;

    absv = abs(v);
    if absv < speed1
        regen = 0;
    elseif absv <= speed2
        regen = 0.95 * (absv-speed1)/dspeed;
    else
        regen = 0.95;
    end

    if SOC <= 0.8
        SOCfactor = 1;
    elseif SOC < 1
        SOCfactor = 1 - (SOC-0.8)/(1-0.8);
    else
        SOCfactor = 0;
    end

    regen = regen * SOCfactor;

    APP = a + b*regen;
    BPP = b * (1-regen);

== matlab function MEEN_432_Proj4Part2_version2025A/Longitudinal Dynamics Body Frame/Electric Motor Drive/Battery/MATLAB Function ==
  data: I_batt input; SOC input; I_batt_clipped output
function I_batt_clipped = fcn(I_batt, SOC)
    if SOC <= 0.1
        I_batt_clipped = 0;
    else
        I_batt_clipped = I_batt;
    end

== matlab function MEEN_432_Proj4Part2_version2025A/Throttle and Braking Logic /MATLAB Function1 ==
  data: regen input; viol output; v input
function viol = fcn(regen, v)
    if v < (5*(1600/3600))
        regen_vio = 0;
        if regen == regen_vio
            viol = 0;
        else
            viol = 1;
        end

    elseif v == (25*(1600/3600))
        regen_vio = 0.95;
        if regen == regen_vio
            viol = 0;
        else
            viol = 1;
        end

    elseif v > (25*(1600/3600))
        regen_vio = 0.95;
        if regen == regen_vio
            viol = 0;
        else
            viol = 1;
        end
    else
        regen_vio = (0.95/20)*v;
        if regen == regen_vio
            viol = 0;
        else
            viol = 1;
        end
    end

%     BRK = BPP * -1;
%     if(BRK >= 0) && (1 >= BRK)
%         viol = 0;
%     else
%         viol = 1;
%     end

== matlab function MEEN_432_Proj4Part2_version2025A/CarLateralKinematicsModelBodyFrame/Tire Slip ==
  data: alpha_r output; vy input; alpha_f output; vx input; delta_f input; omega input; obj input
function [alpha_r, alpha_f]= fcn(vy, vx, delta_f, omega, obj)

if abs(vx) > obj.vx_threshold1
    alpha_f = delta_f - (vy + omega * obj.lf) / vx;
    alpha_r = - (vy - omega * obj.lr) / vx;

else
    alpha_f = 0;
    alpha_r = 0;

end

== matlab function MEEN_432_Proj4Part2_version2025A/Driver/MATLAB Function ==
  data: X input; Y input; e_int input; psi input; omega input; delta_f output; vx output; obj input; e_psi output
function [delta_f, vx, e_psi] = SimplestDriver(X, Y, e_int, psi, omega, obj)
% PID steering using psi_int (integral of heading error) and omega (yaw rate)

% --- track geometry ---
R   = 200;      % radius (m)
Lst = 900;      % straight length (m)
y0  = 0;        % bottom straight
y1  = 400;      % top straight
cy  = 200;      % arc centers' y
cxL = 0;        % left arc center x
cxR = Lst;      % right arc center x

% --- controller parameters ---
% PID on heading: delta = delta_ff + Kp*e_psi + Ki*psi_int - Kd*(omega - omega_ref)
Kp = 10;       % proportional on heading error
Ki = 0;    % integral gain (psi_int already integrates e_psi)
Kd = 0.25;      % derivative gain (on yaw-rate error)
Kv = 5;        % speed-control gain

maxSteer = 30*3.141/180; % [rad] steering saturation
vx = obj.vxd;   % vehicle longitudinal speed

% Defaults
psi_ref   = 0;
kappa_ref = 0;  % desired curvature (+ left, - right)
delta_ff  = 0;  % feed-forward steering

if X > Lst
    vx= 1.4*vx 
    % -------- Right semicircle (center at cxR,cy), CCW from bottom to top --------
    % Tangent heading is phi + pi/2
    phi      = atan2(Y - cy, X - cxR);
    psi_ref  = phi + pi/2;
    kappa_ref = 1/R;  % CCW positive
    
    % Geometric + understeer feed-forward
    delta_ff = 3*((obj.lf + obj.lr)*kappa_ref + obj.understeerCoeff * vx^2);


elseif X < 0
    vx= 2*vx 
    % -------- Left semicircle (center at cxL,cy), CCW from top to bottom --------
    phi      = atan2(Y - cy, X - cxL);
    psi_ref  = phi + pi/2;
    kappa_ref = 1/R;  % CCW positive
    
    delta_ff = 3*((obj.lf + obj.lr)*kappa_ref + obj.understeerCoeff * vx^2);

else
    % -------- Inside rectangle (straights) --------
    vx= 5*vx    
    if abs(Y) <= (y1 - y0)/2
        % Bottom straight: motion +x => heading 0
        psi_ref   = 0;
        kappa_ref = 0;
        delta_ff  = 0;
        e_psi     = wrapToPi(psi_ref - psi);
    else
        % Top straight: motion -x => heading pi (or -pi)
        psi_ref   = pi;
        kappa_ref = 0;
        delta_ff  = 0;
        e_psi     = wrapToPi(psi_ref - psi);
    end
end

% --- heading error (wrapped to [-pi, pi]) ---
e_psi = wrapToPi(psi_ref - psi);
omega_ref = kappa_ref * vx;
% derivative term: use yaw-rate error (omega - omega_ref), subtract to damp
delta_f = delta_ff + Kp*e_psi + Ki*e_int - 3*Kd*(omega - omega_ref);

% --- speed control ---
vx = obj.vxd - Kv*(Kp*e_psi + Ki*e_int - Kd*(omega - omega_ref));

% --- saturation ---
%delta_f = min(max(delta, -maxSteer), maxSteer);



% ---------- helpers ----------
function ang = wrapToPi(ang)
% Wrap any angle to [-pi, pi]
ang = mod(ang + pi, 2*pi) - pi;
end
end

== matlab function MEEN_432_Proj4Part2_version2025A/Subsystem/MATLAB Function ==
  data: X input; calculate_gradient output; Y input
function calculate_gradient = fcn(X, Y)
% Compute gradient of z(X) and apply sign depending on Y

% Ensure X is scalar (adapt for vectors if needed)
t = (X - 450)/50;
z = 10 * exp(t) ./ (1 + exp(t));        % original function

% analytic derivative dz/dX
dzdx = 0.2 * exp(t) ./ (1 + exp(t)).^2;

if X > 0 && X < 900
    if Y < 200
        calculate_gradient =  dzdx;
    elseif Y > 500
        calculate_gradient = -dzdx;
    else
        % define behavior for 200 <= Y <= 500
        calculate_gradient = 0;
    end
else
    calculate_gradient = 0;
end

end

== matlab function MEEN_432_Proj4Part2_version2025A/Longitudinal Dynamics Body Frame/Electric Motor Drive/Electric Motor/MATLAB Function1 ==
  data: Tm input; I_bus output; Wm input; Effm input; V_bus input
function I_bus = fcn(Tm, Wm, Effm, V_bus)
    Pm = Tm*Wm;
    sgn_m = Pm / (abs(Pm) + 0.001);
    Pe = Pm / (Effm^sgn_m);
    if V_bus > 1
        I_bus = Pe/V_bus;
    else
        I_bus = 0;
    end

== matlab function MEEN_432_Proj4Part2_version2025A/Longitudinal Dynamics Body Frame/Wheel /MATLAB Function ==
  data: r_w input; v_w input; omega_w input; lambda output
function lambda = tire_slip_ratio(r_w, v_w, omega_w)
% r_w - wheel radius
% v_w - wheel axle speed (m/s)
% omega_w - wheel speed (rad/s)
% lambda - tire slip ratio

epsilon = 0.0001; % a small number for numerical smoothening

if (r_w * omega_w >= v_w - epsilon)
    lambda = (r_w * omega_w - v_w) / (abs(r_w * omega_w) + epsilon);
else
    lambda = (r_w * omega_w - v_w) / (abs(v_w) + epsilon);
end

== matlab function MEEN_432_Proj4Part2_version2025A/Longitudinal Dynamics Body Frame/Wheel /MATLAB Function1 ==
  data: tau_axle input; alpha_w output; tau_brake input; I_in input; I_w input; r_w input; F_x input
function alpha_w = wheel_acceleration(tau_axle, tau_brake, I_in, I_w, r_w, F_x)
% tau_axle - axle torque (Nm)
% tau_brake - brake torque (Nm)
% I_in - input inertia (Kg m^2)
% I_w - wheel inertia (Kg m^2)
% r_w - tire radius (m)
% F_x - tractive force from tire contact (N)
% alpha_w = wheel (angular) acceleration (rad / s^2)

alpha_w = (tau_axle - tau_brake - F_x * r_w ) / (I_in + I_w);

== matlab function MEEN_432_Proj4Part2_version2025A/Longitudinal Dynamics Body Frame/Wheel /MATLAB Function2 ==
  data: lambda input; F_x output; lambda_max input; nominal_stiffness input; mu input; mass input
function F_x = tire_tractive_force(lambda, lambda_max, nominal_stiffness, mu, mass )
% lambda - tire slip ratio
% lambda_max - maximum tire slip ratio for F_x calculations
% nominal_stiffness - tire long stiffness (N)
% mu - (effective) friction coefficient - in the range [0, 1]
% mass - vehicle mass for normal force calculation

g = 9.81; % gravity - m/ s^2

N = mass * g/4;  % assume 4 tires and equal distribution across tires

C_lambda = nominal_stiffness * mu * N;
if lambda >= 0
    F_x = C_lambda * min(lambda_max, lambda);
else
    F_x = C_lambda * max(-lambda_max, lambda);
end

== matlab function MEEN_432_Proj4Part2_version2025A/Longitudinal Dynamics Body Frame/Electric Motor Drive/Inverter/Inverter Calculations ==
  data: V_bat input; Eff_I input; V_bus output; I_bus input; I_bat output
function [V_bus, I_bat] = fcn(V_bat, Eff_I, I_bus)
    V_bus = V_bat; % Vbus = Vbat * r, where r is the inverter conversion ratio % * I_bat * Eff_I^(sgn_Pbat))/ I_bus;
    P_bus = V_bus *I_bus;
    sgn_Pbus = P_bus / (abs(P_bus) + 0.001);
    
    if V_bat > 1
        I_bat = (P_bus / Eff_I^sgn_Pbus) / V_bat ;
    else
        I_bat = 0;
    end

end

% double check

== matlab function MEEN_432_Proj4Part2_version2025A/CarBodyFrame2InertialFrame/KinematicVehicleModel_derivatives ==
  data: vx input; vy input; psi input size=1; Xdot output; Ydot output
function [Xdot, Ydot] = fcn(vx, vy, psi)
    temp = TF(psi) * [vx;vy]; 
    Xdot = temp(1);
    Ydot = temp(2);
  
end

function y = TF(psi)
    y = [cos(psi), -sin(psi); sin(psi), cos(psi)];
end

== matlab function MEEN_432_Proj4Part2_version2025A/Longitudinal Dynamics Body Frame/Brake System/Brake Torque ==
  data: BBcmd input; Tbcap input; Tb output; w_wheel input
function Tb = fcn(BBcmd, Tbcap, w_wheel)
% DESCRIPTION: 
%   This function takes the brake torque capacity, the angular velocity of
%   the wheel. A simple approximation for the brake torque capacity is 
%   the brake command times some calibratable constant 

% INPUTS:
%   BBcmd - brake percent command
%   Tbcap - brake torque capacity  [N-m]
%   w_wheel - wheels angular velocity [rad/s]

% OUTPUTS:
%   Tb - actual brake torque [N-m]

Tb = -BBcmd * Tbcap * (w_wheel / (abs(w_wheel) + 0.001));

end

== matlab function MEEN_432_Proj4Part2_version2025A/CarLateralKinematicsModelBodyFrame/Lateral Dynamics ==
  data: Fyr input; ay output; Fyf input; vx input; omega input; omega_dot output; obj input
function [ay, omega_dot]= fcn(Fyr, Fyf, vx, omega, obj)

ay = -vx * omega + (Fyf + Fyr)/obj.Mass;

omega_dot = (Fyf*obj.lf - Fyr*obj.lr)/obj.Inertia;

end
